simulink model "sampleModel72"  (R2021b)
settings: Solver=VariableStepAuto  StartTime=0.0  StopTime=10.0  RelTol=1e-3
undefined symbols (not defined in the file or in its folder): Newton, Raphson
libraries: simulink x4, slpidlib x1
settings Model: Creator=user  LastModifiedBy=user

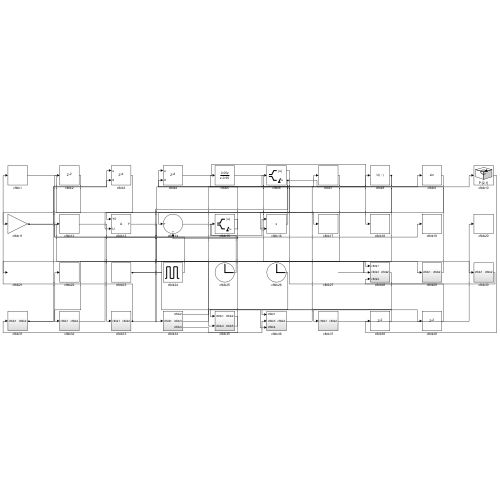
[thumbnail: Simulink's stored preview of the top-level diagram]
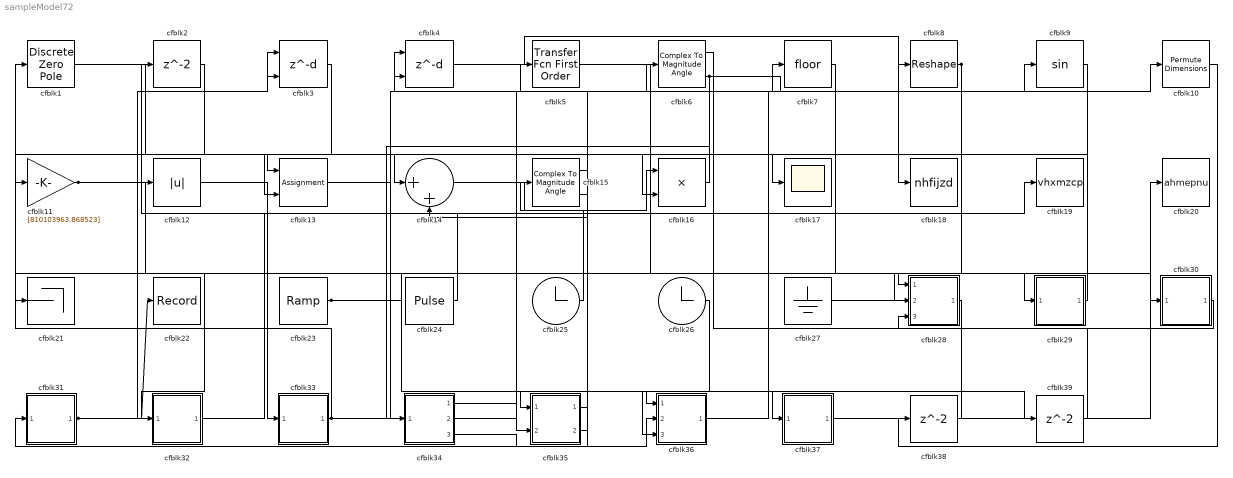
== system sampleModel72 ==
  cfblk1 : DiscreteZeroPole  Poles=[0 0.5]  Gain=1
  cfblk10 : PermuteDimensions
  cfblk11 : Gain  Gain=[810103963.868523]
  cfblk12 : Abs
  cfblk13 : Assignment  DiagnosticForDimensions=Warning  IndexOptions=Index vector (dialog)  Indices=1  OutputSizes=1
  cfblk14 : Sum  Inputs=|++
  cfblk15 : ComplexToMagnitudeAngle
  cfblk16 : Product  Inputs=**
  cfblk17 : Scope
  cfblk18 : ToWorkspace  VariableName=nhfijzd  SaveFormat=Timeseries  SampleTime=-1
  cfblk19 : ToWorkspace  VariableName=vhxmzcp  SaveFormat=Timeseries  SampleTime=-1
  cfblk2 : Delay  SampleTime=1
  cfblk20 : ToWorkspace  VariableName=ahmepnu  SaveFormat=Timeseries  SampleTime=-1
  cfblk21 : Terminator
  cfblk22 : Record  FileSettingsInternal="{\"entries\":[{\"content\":{\"excelSettings\":{\"content\":{},\"type\":\"Streamout.ExcelSettings\"}},\"type\":\"Streamout.FileSettingStorage\",\"uuid\":\"193b0c55-366d-49de-a14d-0c217ef1c26d\"}],\"packageUris\":[\"http://schema.mathworks.com/mf0/streamout_blocks/R2020a\"],\"version\":\"1.0\"}"  SignalsInternal="{\"entries\":[{\"content\":{\"signals\":[{\"content\":{\"blockPath\":[\"sampleModel72/cfblk22\"],\"channel\":[],\"dimensions\":[1],\"domain\":\"sampleModel72/cfblk22\",\"lineColor\":\"#b746ff\",\"plots\":[1],\"port\":1,\"sid\":[\"\"],\"signalID\":2693,\"signalName\":\"cfblk31\"},\"type\":\"RecordBlkView.Signal\",\"uuid\":\"b1c63b00-41fe-450c-99aa-0a25e93ed43c\"}]},\"type\":\"RecordBlkView.InputSignals\",\"uuid\":\"c236b533-25b0-4c56-a71d-1c2f69872e99\"}],\"packageUris\":[\"http://schema.mathworks.com/mf0/streamout_blocks/R2020a\"],\"version\":\"1.0\"}"  VisualizationBindings="{\"sparklinesplugin\":{\"info\":[{\"bindingParametersList\":[],\"subplotID\":1}]}}"
  cfblk23 : simulink/Sources/Ramp  slope=[-7181.517370]  start=[17.868118]  InitialOutput=[-709348.513331]
  cfblk24 : DiscretePulseGenerator  PulseType=Time based  Amplitude=[-23157053.221700]  Period=[46985046.531968]  PulseWidth=5  PhaseDelay=[8.000000]
  cfblk25 : Clock
  cfblk26 : Clock
  cfblk27 : Ground
  cfblk28 : Subsystem
  cfblk29 : Subsystem
  cfblk3 : Delay  DelayLengthSource=Input port  SampleTime=1
      settings: InputPortMap=u0,p1
  cfblk30 : Subsystem
  cfblk31 : Subsystem
  cfblk32 : Subsystem
  cfblk33 : Subsystem
  cfblk34 : Subsystem
  cfblk35 : Subsystem
  cfblk36 : Subsystem
  cfblk37 : Subsystem
  cfblk38 : Delay  SampleTime=1
  cfblk39 : Delay  SampleTime=1
  cfblk4 : Delay  DelayLengthSource=Input port  SampleTime=1
      settings: InputPortMap=u0,p1
  cfblk5 : simulink/Discrete/Transfer Fcn First Order  PoleZ=0.95  ICPrevOutput=0.0  DoSatur=off
  cfblk6 : ComplexToMagnitudeAngle
  cfblk7 : Rounding
  cfblk8 : Reshape
  cfblk9 : Trigonometry
  wires:
  cfblk3/1 -> cfblk13/1
  cfblk37/1(cfblk2) -> cfblk20/1
  cfblk6/1 -> cfblk14/1
  cfblk6/2 -> cfblk34/1(cfblk1), cfblk8/1
  cfblk33/1(cfblk2) -> cfblk1/1, cfblk10/1
  cfblk28/1(cfblk2) -> cfblk37/1(cfblk1)
  cfblk23/1 -> cfblk28/1(cfblk1), cfblk36/3(cfblk4)
  cfblk4/1 -> cfblk18/1
  cfblk31/1(cfblk2) -> cfblk22/1, cfblk3/2
  cfblk5/1 -> cfblk30/1(cfblk1)
  cfblk12/1 -> cfblk33/1(cfblk1)
  cfblk36/1(cfblk2) -> cfblk9/1
  cfblk29/1(cfblk2) -> cfblk4/1
  cfblk2/1 -> cfblk11/1
  cfblk26/1 -> cfblk36/1(cfblk1)
  cfblk35/1(cfblk2) -> cfblk31/1(cfblk1)
  cfblk1/1 -> cfblk17/1
  cfblk9/1 -> cfblk13/2
  cfblk14/1 -> cfblk16/1
  cfblk32/1(cfblk2) -> cfblk19/1
  cfblk13/1 -> cfblk28/2(cfblk3)
  cfblk7/1 -> cfblk21/1
  cfblk27/1 -> cfblk29/1(cfblk1)
  cfblk24/1 -> cfblk2/1
  cfblk11/1 -> cfblk35/2(cfblk4), cfblk3/1
  cfblk30/1(cfblk2) -> cfblk28/3(cfblk4)
  cfblk8/1 -> cfblk32/1(cfblk1), cfblk16/2
  cfblk16/1 -> cfblk4/2
  cfblk35/2(cfblk5) -> cfblk12/1
  cfblk15/1 -> cfblk14/2
  cfblk25/1 -> cfblk15/1
  cfblk34/2(cfblk3) -> cfblk7/1
  cfblk15/2 -> cfblk5/1
  cfblk34/3(cfblk4) -> cfblk36/2(cfblk3)
  cfblk10/1 -> cfblk38/1
  cfblk38/1 -> cfblk35/1(cfblk1)
  cfblk34/1(cfblk2) -> cfblk39/1
  cfblk39/1 -> cfblk6/1

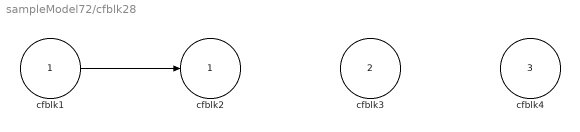
== system sampleModel72/cfblk28 ==
  cfblk1 : Inport
  cfblk3 : Inport  Port=2
  cfblk4 : Inport  Port=3
  cfblk2 : Outport
  wires:
  cfblk1/1 -> cfblk2/1

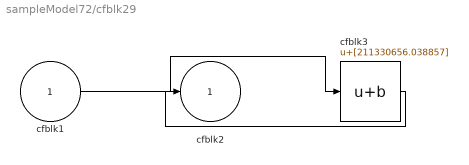
== system sampleModel72/cfblk29 ==
  cfblk1 : Inport
  cfblk3 : Bias  Bias=[211330656.038857]
  cfblk2 : Outport
  wires:
  cfblk1/1 -> cfblk3/1
  cfblk3/1 -> cfblk2/1

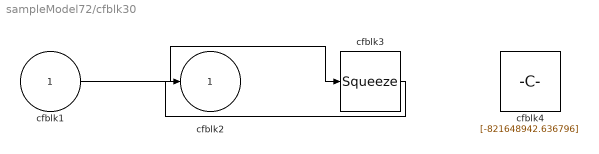
== system sampleModel72/cfblk30 ==
  cfblk1 : Inport
  cfblk3 : Squeeze
  cfblk4 : Constant  Value=[-821648942.636796]  SampleTime=1
  cfblk2 : Outport
  wires:
  cfblk1/1 -> cfblk3/1
  cfblk3/1 -> cfblk2/1

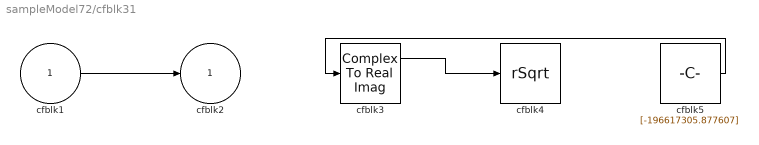
== system sampleModel72/cfblk31 ==
  cfblk1 : Inport
  cfblk3 : ComplexToRealImag
  cfblk4 : Sqrt  Operator=rSqrt  AlgorithmType=Newton-Raphson  SaturateOnIntegerOverflow=on
  cfblk5 : Constant  Value=[-196617305.877607]  SampleTime=1
  cfblk2 : Outport
  wires:
  cfblk3/1 -> cfblk4/1
  cfblk1/1 -> cfblk2/1
  cfblk5/1 -> cfblk3/1

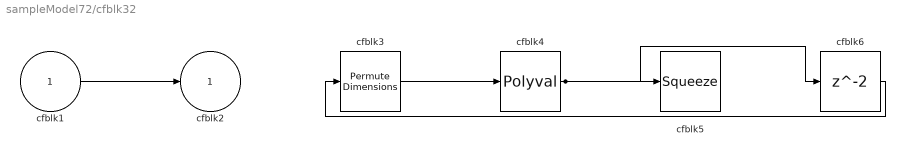
== system sampleModel72/cfblk32 ==
  cfblk1 : Inport
  cfblk3 : PermuteDimensions
  cfblk4 : Polyval  Coefs=[ +2.081618890e-019, -1.441693666e-014, +4.719686976e-010, -8.536869453e-006, +1.621573104e-001, -8.087801117e+001 ]
  cfblk5 : Squeeze
  cfblk6 : Delay  SampleTime=1
  cfblk2 : Outport
  wires:
  cfblk3/1 -> cfblk4/1
  cfblk1/1 -> cfblk2/1
  cfblk4/1 -> cfblk5/1, cfblk6/1
  cfblk6/1 -> cfblk3/1

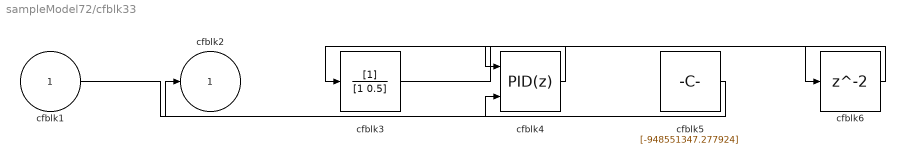
== system sampleModel72/cfblk33 ==
  cfblk1 : Inport
  cfblk3 : DiscreteFilter  SampleTime=1
  cfblk4 : slpidlib/PID Controller (2DOF)  Controller=PID  Form=Parallel  TimeDomain=Discrete-time  UseExternalTs=off  SampleTime=1  IntegratorMethod=Forward Euler  FilterMethod=Forward Euler  ControllerParametersSource=internal  P=1  I=1  D=0  UseFilter=on  N=100  b=1  c=1  TunerSelectOption=Transfer Function Based (PID Tuner App)  InitialConditionSource=internal  InitialConditionForIntegrator=0  InitialConditionForFilter=0  DifferentiatorICPrevScaledInput=0  ExternalReset=none  TrackingMode=off  Kt=1  LimitOutput=off  SatLimitsSource=internal  UpperSaturationLimit=inf  LowerSaturationLimit=-inf  LinearizeAsGain=off  AntiWindupMode=none  Kb=1  POutMin=[]  POutMax=[]  IOutMin=[]  IOutMax=[]  DOutMin=[]  DOutMax=[]  NOutMin=[]  NOutMax=[]  bOutMin=[]  bOutMax=[]  cOutMin=[]  cOutMax=[]  SumOutMin=[]  SumOutMax=[]  SaturationOutMin=[]  SaturationOutMax=[]  PParamMin=[]  PParamMax=[]  IParamMin=[]  IParamMax=[]  DParamMin=[]  DParamMax=[]  NParamMin=[]  NParamMax=[]  bParamMin=[]  bParamMax=[]  cParamMin=[]  cParamMax=[]  KbParamMin=[]  KbParamMax=[]  KtParamMin=[]  KtParamMax=[]  KbOutMin=[]  KbOutMax=[]  KtOutMin=[]  KtOutMax=[]  IntegratorOutMin=[]  IntegratorOutMax=[]  FilterOutMin=[]  FilterOutMax=[]  SumI1OutMin=[]  SumI1OutMax=[]  SumI2OutMin=[]  SumI2OutMax=[]  SumI3OutMin=[]  SumI3OutMax=[]  SumI4OutMin=[]  SumI4OutMax=[]  SumDOutMin=[]  SumDOutMax=[]  Sum1OutMin=[]  Sum1OutMax=[]  Sum2OutMin=[]  Sum2OutMax=[]  Sum3OutMin=[]  Sum3OutMax=[]  DifferentiatorOutMin=[]  DifferentiatorOutMax=[]  FilterDiffOutCoefMin=[]  FilterDiffOutCoefMax=[]  ReciprocalOutMin=[]  ReciprocalOutMax=[]  SumDenOutMin=[]  SumDenOutMax=[]  SumNumOutMin=[]  SumNumOutMax=[]  DivideOutMin=[]  DivideOutMax=[]  UdiffTsProdOutMin=[]  UdiffTsProdOutMax=[]  NTsProdOutMin=[]  NTsProdOutMax=[]  UintegralTsProdOutMin=[]  UintegralTsProdOutMax=[]  UngainTsProdOutMin=[]  UngainTsProdOutMax=[]  IntegratorContinuousStateAttributes=''  IntegratorStateMustResolveToSignalObject=off  IntegratorRTWStateStorageClass=Auto  FilterContinuousStateAttributes=''  FilterStateMustResolveToSignalObject=off  FilterRTWStateStorageClass=Auto  ParallelPVariant=InternalParameters  IdealPVariant=Disabled  IVariant=InternalParameters  DVariant=InternalParameters  bVariant=InternalParameters  cVariant=InternalParameters  IntegratorVariant=Discrete  SatVariant=Disabled  AWVariant=Passthrough  PCopyVariant=Disabled  TRVariant=Disabled  FdbkBlocksVariant=Forward  IdealPFdbkVariant=Disabled  SatFdbkVariant=Disabled  DerivativeFilterVariant=ForwardEulerFilter  NVariant=InternalParameters  NCopyVariant=Disabled  FilterICVariant=InternalICsFilter  IntegratorICVariant=InternalICs  ExternalResetVariant=Disabled  TRSumVariant=Passthrough  SumFdbkVariant=Disabled  SumVariant=Sum_PID  TsampFilterVariant=InternalTs  TsampNgainVariant=Passthrough  TsampIntegralVariant=Passthrough  ExternalSaturationOutDataTypeStr=Inherit: Same as second input
      settings: SourceProductBaseCode=SL
  cfblk5 : Constant  Value=[-948551347.277924]  SampleTime=1
  cfblk6 : Delay  SampleTime=1
  cfblk2 : Outport
  wires:
  cfblk4/1 -> cfblk3/1
  cfblk5/1 -> cfblk2/1
  cfblk1/1 -> cfblk4/2
  cfblk3/1 -> cfblk6/1
  cfblk6/1 -> cfblk4/1

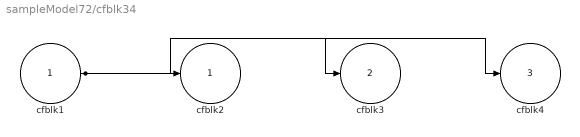
== system sampleModel72/cfblk34 ==
  cfblk1 : Inport
  cfblk2 : Outport
  cfblk3 : Outport  Port=2
  cfblk4 : Outport  Port=3
  wires:
  cfblk1/1 -> cfblk3/1, cfblk4/1, cfblk2/1

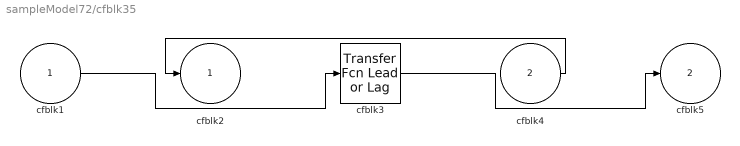
== system sampleModel72/cfblk35 ==
  cfblk1 : Inport
  cfblk4 : Inport  Port=2
  cfblk3 : simulink/Discrete/Transfer Fcn Lead or Lag  PoleZ=0.95  ZeroZ=0.75  ICPrevOutput=0.0  ICPrevInput=0.0  DoSatur=off
      settings: SourceProductBaseCode=SL
  cfblk2 : Outport
  cfblk5 : Outport  Port=2
  wires:
  cfblk4/1 -> cfblk2/1
  cfblk1/1 -> cfblk3/1
  cfblk3/1 -> cfblk5/1

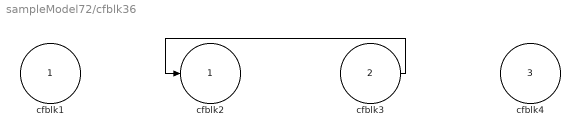
== system sampleModel72/cfblk36 ==
  cfblk1 : Inport
  cfblk3 : Inport  Port=2
  cfblk4 : Inport  Port=3
  cfblk2 : Outport
  wires:
  cfblk3/1 -> cfblk2/1

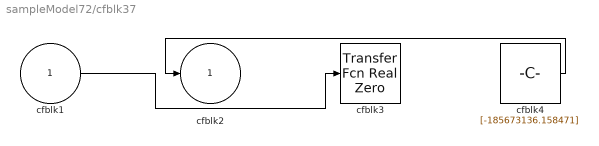
== system sampleModel72/cfblk37 ==
  cfblk1 : Inport
  cfblk3 : simulink/Discrete/Transfer Fcn Real Zero  ZeroZ=0.75  ICPrevInput=0.0  DoSatur=off
      settings: SourceProductBaseCode=SL
  cfblk4 : Constant  Value=[-185673136.158471]  SampleTime=1
  cfblk2 : Outport
  wires:
  cfblk4/1 -> cfblk2/1
  cfblk1/1 -> cfblk3/1
